simulink library "jud"  (Simulink 8.2)
settings: Solver=ode45  StartTime=0.0  StopTime=10.0  RelTol=1e-3
undefined symbols (not defined in the file or in its folder): ENUM_EPSADASABREASON_GEAR_POSITION_ERROR, ENUM_EPSADASABREASON_THERMAL_ERROR, ENUM_EPSADASABREASON_VEHICLE_SPEED_ERROR, ENUM_EPSLFCSTATUS_NOTAVAIL_PERM, ENUM_EPSLFCSTATUS_NOTAVAIL_TEMP, ENUM_EPSLFCSTATUS_OFF, ENUM_EPSLFCSTATUS_READY, ENUM_EPSLFCSTATUS_TRANSITION, ENUM_EPSLKASTATUS_NOTAVAIL_PERM, ENUM_EPSLKASTATUS_NOTAVAIL_TEMP, ENUM_EPSLKASTATUS_OFF, ENUM_EPSLKASTATUS_READY, ENUM_HMISTATE_ACTIVE, ENUM_KEYSWITCH_ON, ENUM_LFCSTATE_AUTOSTEERING, ENUM_LFCSTATE_STANDBY, ENUM_SENSORSTATE_NORMAL, FALSE, KAPP_VehicleWidth_m, KJUD_EPSLimition_kph, KJUD_EPSLimitionHysis_kph, KJUD_LFC4StandbyDelay_s, KJUD_SoftenTimerThr_s, TRUE, VJUD_LFCOffCount4LKAStandby_s, VJUD_LKAReActingDelay_s, VJUD_TLCTriggerReActingDelay_s
libraries: hcu_lib x12, simulink x10, jcc x1, jcw x1, jeb x1
(part 1 of 3)
settings Model: Creator=xsellart  LastModifiedBy=13192

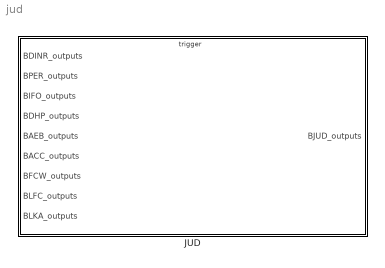
== system jud ==
  JUD : Subsystem

== system jud/JUD ==
  BDINR_outputs : Inport  OutDataTypeStr=Bus: BDINR_outputs
  BPER_outputs : Inport  Port=2  OutDataTypeStr=Bus: BPER_outputs
  BIFO_outputs : Inport  Port=3  OutDataTypeStr=Bus: BIFO_outputs
  BDHP_outputs : Inport  Port=4  OutDataTypeStr=Bus: BDHP_outputs
  BAEB_outputs : Inport  Port=5  OutDataTypeStr=Bus: BAEB_outputs
  BACC_outputs : Inport  Port=6  OutDataTypeStr=Bus: BACC_outputs
  BFCW_outputs : Inport  Port=7  OutDataTypeStr=Bus: BFCW_outputs
  BLFC_outputs : Inport  Port=8  OutDataTypeStr=Bus: BLFC_outputs
  BLKA_outputs : Inport  Port=9  OutDataTypeStr=Bus: BLKA_outputs
  trig_JUD : TriggerPort  TriggerType=function-call
      settings: AttributesFormatString=State = %<StatesWhenEnabling>
  Bus Creator : BusCreator  Inputs=61  OutDataTypeStr=Bus: BJUD_outputs
  jud : Subsystem
  BJUD_outputs : Outport  OutDataTypeStr=Bus: BJUD_outputs
  wires:
  Bus Creator/1 -> BJUD_outputs/1  "BJUD_outputs"
  BDINR_outputs/1 -> jud/1(BDINR_outputs)
  BPER_outputs/1 -> jud/2(BPER_outputs)
  BIFO_outputs/1 -> jud/3(BIFO_outputs)
  BDHP_outputs/1 -> jud/4(BDHP_outputs)
  BAEB_outputs/1 -> jud/5(BAEB_outputs)
  BACC_outputs/1 -> jud/6(BACC_outputs)
  BFCW_outputs/1 -> jud/7(BFCW_outputs)
  jud/1(VJUD_FCWEnableReq_flg) -> Bus Creator/1
  jud/2(VJUD_FCWOperational_flg) -> Bus Creator/2
  jud/8(VJUD_AEBEnableReq_flg) -> Bus Creator/8
  jud/41(VJUD_LKALeftActionReq_flg) -> Bus Creator/41
  jud/12(VJUD_AEBReturnOperational_flg) -> Bus Creator/12
  jud/31(VJUD_LFCTempFailureReq_flg) -> Bus Creator/31
  jud/10(VJUD_AEBSpeedInRange_flg) -> Bus Creator/10
  jud/20(VJUD_ACCOverrideReq_flg) -> Bus Creator/20
  jud/13(VJUD_AEBAutoBraking_flg) -> Bus Creator/13
  jud/11(VJUD_AEBActionReq_flg) -> Bus Creator/11
  jud/21(VJUD_ACCSetSpeed_kph) -> Bus Creator/21
  jud/34(VJUD_DegradedToAutoStr_flg) -> Bus Creator/34
  jud/44(VJUD_LKANoADASFailure_flg) -> Bus Creator/44
  jud/49(VJUD_LKATempFailureRecover_flg) -> Bus Creator/49
  jud/28(VJUD_LFCActionReq_flg) -> Bus Creator/28
  jud/33(VJUD_LFCOffRecover_flg) -> Bus Creator/33
  jud/42(VJUD_LKARightActionReq_flg) -> Bus Creator/42
  jud/29(VJUD_LFCDegradedReq_flg) -> Bus Creator/29
  jud/3(VJUD_FCWSpeedInRange_flg) -> Bus Creator/3
  jud/16(VJUD_ACCActiveReq_flg) -> Bus Creator/16
  jud/45(VJUD_LKAOffRecover_flg) -> Bus Creator/45
  jud/14(VJUD_AEBDeactivationReq_flg) -> Bus Creator/14
  jud/30(VJUD_LFCSoftenReq_flg) -> Bus Creator/30
  jud/26(VJUD_LFCCheckNormalFailure_flg) -> Bus Creator/26
  jud/15(VJUD_ACCEnableReq_flg) -> Bus Creator/15
  jud/7(VJUD_FCWDBSAllowed_flg) -> Bus Creator/7
  jud/47(VJUD_LKALeftOperationalRecover_flg) -> Bus Creator/47
  jud/24(VJUD_ACCSetSpeedSel_flg) -> Bus Creator/24
  jud/40(VJUD_LKAOperationalReq_flg) -> Bus Creator/40
  jud/5(VJUD_FCWReturnOperational_flg) -> Bus Creator/5
  jud/27(VJUD_LFCEnabledReq_flg) -> Bus Creator/27
  jud/43(VJUD_LKATempFailureReq_flg) -> Bus Creator/43
  jud/37(VJUD_LKACheckNormal_flg) -> Bus Creator/37
  jud/9(VJUD_AEBOperational_flg) -> Bus Creator/9
  jud/25(VJUD_LFCCheckNormal_flg) -> Bus Creator/25
  jud/39(VJUD_LKAEnabledReq_flg) -> Bus Creator/39
  jud/23(VJUD_ACCHMISelTimeGap_s) -> Bus Creator/23
  jud/17(VJUD_ACCDeactivationReq_flg) -> Bus Creator/17
  jud/36(VJUD_SoftenTimeThr_s) -> Bus Creator/36
  jud/46(VJUD_LKAStandbyRecover_flg) -> Bus Creator/46
  jud/4(VJUD_FCWActionReq_flg) -> Bus Creator/4
  jud/48(VJUD_LKARightOperationalRecover_flg) -> Bus Creator/48
  jud/22(VJUD_ACCSetTimeGap_s) -> Bus Creator/22
  jud/32(VJUD_LFCNoADASFailure_flg) -> Bus Creator/32
  jud/35(VJUD_LFCTempFailureRecover_flg) -> Bus Creator/35
  jud/18(VJUD_ACCStandstillReq_flg) -> Bus Creator/18
  jud/19(VJUD_ACCRefollowReq_flg) -> Bus Creator/19
  jud/38(VJUD_LKACheckNormalFailure_flg) -> Bus Creator/38
  BLFC_outputs/1 -> jud/8(BLFC_outputs)
  BLKA_outputs/1 -> jud/9(BLKA_outputs)
  jud/50(VJUD_LCACheckNormal_flg) -> Bus Creator/50
  jud/57(VJUD_LCAOffRecover_flg) -> Bus Creator/57
  jud/51(VJUD_LCAEnabledReq_flg) -> Bus Creator/51
  jud/56(VJUD_LCANoADASFailure_flg) -> Bus Creator/56
  jud/55(VJUD_LCATempFailureReq_flg) -> Bus Creator/55
  jud/58(VJUD_LCAStandbyRecover_flg) -> Bus Creator/58
  jud/59(VJUD_LCALeftOperationalRecover_flg) -> Bus Creator/59
  jud/52(VJUD_LCAOperationalReq_flg) -> Bus Creator/52
  jud/61(VJUD_LCATempFailureRecover_flg) -> Bus Creator/61
  jud/60(VJUD_LCARightOperationalRecover_flg) -> Bus Creator/60
  jud/53(VJUD_LCALeftActionReq_flg) -> Bus Creator/53
  jud/54(VJUD_LCARightActionReq_flg) -> Bus Creator/54
  jud/6(VJUD_FCWDeactivationReq_flg) -> Bus Creator/6

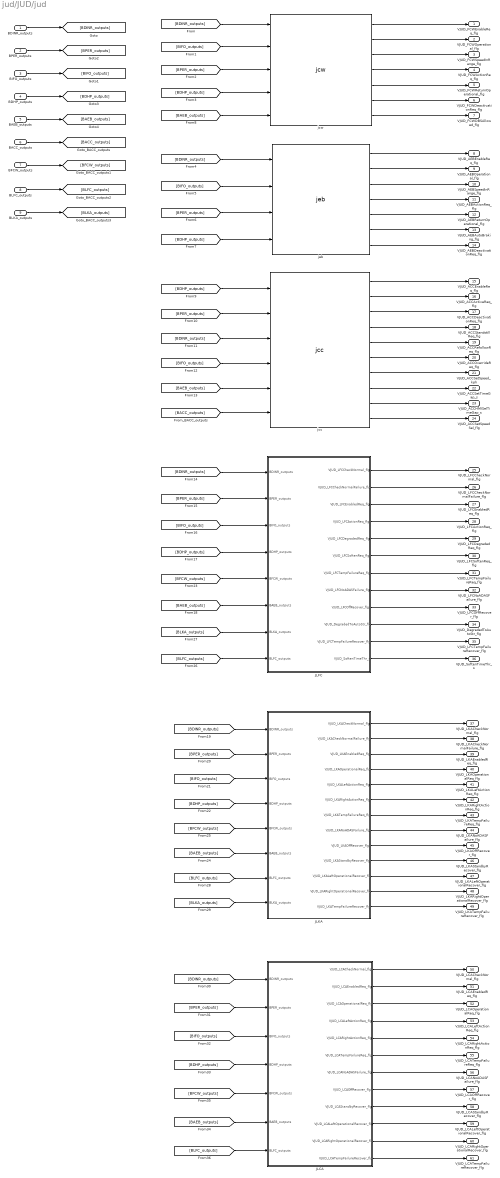
== system jud/JUD/jud ==
  BDINR_outputs : Inport  OutDataTypeStr=Bus: BDINR_outputs
  BPER_outputs : Inport  Port=2  OutDataTypeStr=Bus: BPER_outputs
  BIFO_outputs : Inport  Port=3  OutDataTypeStr=Bus: BIFO_outputs
  BDHP_outputs : Inport  Port=4  OutDataTypeStr=Bus: BDHP_outputs
  BAEB_outputs : Inport  Port=5  OutDataTypeStr=Bus: BAEB_outputs
  BACC_outputs : Inport  Port=6  OutDataTypeStr=Bus: BACC_outputs
  BFCW_outputs : Inport  Port=7  OutDataTypeStr=Bus: BFCW_outputs
  BLFC_outputs : Inport  Port=8  OutDataTypeStr=Bus: BLFC_outputs
  BLKA_outputs : Inport  Port=9  OutDataTypeStr=Bus: BLKA_outputs
  JLCA : Subsystem
  JLFC : Subsystem
  JLKA : Subsystem
  jcc : jcc/jcc
  jcw : jcw/jcw
  jeb : jeb/jeb
  VJUD_FCWEnableReq_flg : Outport
  VJUD_FCWOperational_flg : Outport  Port=2
  VJUD_FCWSpeedInRange_flg : Outport  Port=3
  VJUD_FCWActionReq_flg : Outport  Port=4
  VJUD_FCWReturnOperational_flg : Outport  Port=5
  VJUD_FCWDeactivationReq_flg : Outport  Port=6
  VJUD_FCWDBSAllowed_flg : Outport  Port=7
  VJUD_AEBEnableReq_flg : Outport  Port=8
  VJUD_AEBOperational_flg : Outport  Port=9
  VJUD_AEBSpeedInRange_flg : Outport  Port=10
  VJUD_AEBActionReq_flg : Outport  Port=11
  VJUD_AEBReturnOperational_flg : Outport  Port=12
  VJUD_AEBAutoBraking_flg : Outport  Port=13
  VJUD_AEBDeactivationReq_flg : Outport  Port=14
  VJUD_ACCEnableReq_flg : Outport  Port=15
  VJUD_ACCActiveReq_flg : Outport  Port=16
  VJUD_ACCDeactivationReq_flg : Outport  Port=17
  VJUD_ACCStandstillReq_flg : Outport  Port=18
  VJUD_ACCRefollowReq_flg : Outport  Port=19
  VJUD_ACCOverrideReq_flg : Outport  Port=20
  VJUD_ACCSetSpeed_kph : Outport  Port=21
  VJUD_ACCSetTimeGap_s : Outport  Port=22
  VJUD_ACCHMISelTimeGap_s : Outport  Port=23
  VJUD_ACCSetSpeedSel_flg : Outport  Port=24
  VJUD_LFCCheckNormal_flg : Outport  Port=25
  VJUD_LFCCheckNormalFailure_flg : Outport  Port=26
  VJUD_LFCEnabledReq_flg : Outport  Port=27
  VJUD_LFCActionReq_flg : Outport  Port=28
  VJUD_LFCDegradedReq_flg : Outport  Port=29
  VJUD_LFCSoftenReq_flg : Outport  Port=30
  VJUD_LFCTempFailureReq_flg : Outport  Port=31
  VJUD_LFCNoADASFailure_flg : Outport  Port=32
  VJUD_LFCOffRecover_flg : Outport  Port=33
  VJUD_DegradedToAutoStr_flg : Outport  Port=34
  VJUD_LFCTempFailureRecover_flg : Outport  Port=35
  VJUD_SoftenTimeThr_s : Outport  Port=36
  VJUD_LKACheckNormal_flg : Outport  Port=37
  VJUD_LKACheckNormalFailure_flg : Outport  Port=38
  VJUD_LKAEnabledReq_flg : Outport  Port=39
  VJUD_LKAOperationalReq_flg : Outport  Port=40
  VJUD_LKALeftActionReq_flg : Outport  Port=41
  VJUD_LKARightActionReq_flg : Outport  Port=42
  VJUD_LKATempFailureReq_flg : Outport  Port=43
  VJUD_LKANoADASFailure_flg : Outport  Port=44
  VJUD_LKAOffRecover_flg : Outport  Port=45
  VJUD_LKAStandbyRecover_flg : Outport  Port=46
  VJUD_LKALeftOperationalRecover_flg : Outport  Port=47
  VJUD_LKARightOperationalRecover_flg : Outport  Port=48
  VJUD_LKATempFailureRecover_flg : Outport  Port=49
  VJUD_LCACheckNormal_flg : Outport  Port=50
  VJUD_LCAEnabledReq_flg : Outport  Port=51
  VJUD_LCAOperationalReq_flg : Outport  Port=52
  VJUD_LCALeftActionReq_flg : Outport  Port=53
  VJUD_LCARightActionReq_flg : Outport  Port=54
  VJUD_LCATempFailureReq_flg : Outport  Port=55
  VJUD_LCANoADASFailure_flg : Outport  Port=56
  VJUD_LCAOffRecover_flg : Outport  Port=57
  VJUD_LCAStandbyRecover_flg : Outport  Port=58
  VJUD_LCALeftOperationalRecover_flg : Outport  Port=59
  VJUD_LCARightOperationalRecover_flg : Outport  Port=60
  VJUD_LCATempFailureRecover_flg : Outport  Port=61
  wires:
  [BIFO_outputs] -> jcw/2
  jeb/1 -> VJUD_AEBEnableReq_flg/1
  [BPER_outputs] -> jcw/3
  jcw/1 -> VJUD_FCWEnableReq_flg/1
  jcw/7 -> VJUD_FCWDBSAllowed_flg/1
  [BIFO_outputs] -> jeb/2
  [BDINR_outputs] -> jeb/1
  BPER_outputs/1 -> [BPER_outputs]
  jcw/6 -> VJUD_FCWDeactivationReq_flg/1
  jeb/6 -> VJUD_AEBAutoBraking_flg/1
  BIFO_outputs/1 -> [BIFO_outputs]
  BDHP_outputs/1 -> [BDHP_outputs]
  jcw/4 -> VJUD_FCWActionReq_flg/1
  [BDHP_outputs] -> jcw/4
  jcw/2 -> VJUD_FCWOperational_flg/1
  [BDHP_outputs] -> jeb/4
  jcw/3 -> VJUD_FCWSpeedInRange_flg/1
  jeb/4 -> VJUD_AEBActionReq_flg/1
  [BDINR_outputs] -> jcw/1
  [BPER_outputs] -> jeb/3
  BDINR_outputs/1 -> [BDINR_outputs]
  jeb/7 -> VJUD_AEBDeactivationReq_flg/1
  BAEB_outputs/1 -> [BAEB_outputs]
  [BAEB_outputs] -> jcw/5
  jeb/2 -> VJUD_AEBOperational_flg/1
  jeb/3 -> VJUD_AEBSpeedInRange_flg/1
  jcw/5 -> VJUD_FCWReturnOperational_flg/1
  jeb/5 -> VJUD_AEBReturnOperational_flg/1
  jcc/2 -> VJUD_ACCActiveReq_flg/1
  jcc/3 -> VJUD_ACCDeactivationReq_flg/1
  jcc/1 -> VJUD_ACCEnableReq_flg/1
  jcc/4 -> VJUD_ACCStandstillReq_flg/1
  jcc/5 -> VJUD_ACCRefollowReq_flg/1
  jcc/6 -> VJUD_ACCOverrideReq_flg/1
  jcc/7 -> VJUD_ACCSetSpeed_kph/1
  jcc/8 -> VJUD_ACCSetTimeGap_s/1
  jcc/10 -> VJUD_ACCSetSpeedSel_flg/1
  [BDHP_outputs] -> jcc/1
  [BPER_outputs] -> jcc/2
  [BDINR_outputs] -> jcc/3
  [BIFO_outputs] -> jcc/4
  [BAEB_outputs] -> jcc/5
  BACC_outputs/1 -> [BACC_outputs]
  [BACC_outputs] -> jcc/6
  jcc/9 -> VJUD_ACCHMISelTimeGap_s/1
  JLFC/1(VJUD_LFCCheckNormal_flg) -> VJUD_LFCCheckNormal_flg/1
  JLFC/2(VJUD_LFCCheckNormalFailure_flg) -> VJUD_LFCCheckNormalFailure_flg/1
  JLFC/3(VJUD_LFCEnabledReq_flg) -> VJUD_LFCEnabledReq_flg/1
  JLFC/4(VJUD_LFCActionReq_flg) -> VJUD_LFCActionReq_flg/1
  JLFC/5(VJUD_LFCDegradedReq_flg) -> VJUD_LFCDegradedReq_flg/1
  JLFC/6(VJUD_LFCSoftenReq_flg) -> VJUD_LFCSoftenReq_flg/1
  JLFC/7(VJUD_LFCTempFailureReq_flg) -> VJUD_LFCTempFailureReq_flg/1
  JLFC/8(VJUD_LFCNoADASFailure_flg) -> VJUD_LFCNoADASFailure_flg/1
  JLFC/9(VJUD_LFCOffRecover_flg) -> VJUD_LFCOffRecover_flg/1
  JLFC/10(VJUD_DegradedToAutoStr_flg) -> VJUD_DegradedToAutoStr_flg/1
  JLFC/11(VJUD_LFCTempFailureRecover_flg) -> VJUD_LFCTempFailureRecover_flg/1
  JLFC/12(VJUD_SoftenTimeThr_s) -> VJUD_SoftenTimeThr_s/1
  [BDINR_outputs] -> JLFC/1(BDINR_outputs)
  [BPER_outputs] -> JLFC/2(BPER_outputs)
  [BIFO_outputs] -> JLFC/3(BIFO_outputs)
  [BDHP_outputs] -> JLFC/4(BDHP_outputs)
  [BAEB_outputs] -> JLFC/6(BAEB_outputs)
  BFCW_outputs/1 -> [BFCW_outputs]
  [BPER_outputs] -> JLKA/2(BPER_outputs)
  [BDINR_outputs] -> JLKA/1(BDINR_outputs)
  [BIFO_outputs] -> JLKA/3(BIFO_outputs)
  [BDHP_outputs] -> JLKA/4(BDHP_outputs)
  [BFCW_outputs] -> JLFC/5(BFCW_outputs)
  [BAEB_outputs] -> JLKA/6(BAEB_outputs)
  [BFCW_outputs] -> JLKA/5(BFCW_outputs)
  JLKA/1(VJUD_LKACheckNormal_flg) -> VJUD_LKACheckNormal_flg/1
  JLKA/2(VJUD_LKACheckNormalFailure_flg) -> VJUD_LKACheckNormalFailure_flg/1
  JLKA/3(VJUD_LKAEnabledReq_flg) -> VJUD_LKAEnabledReq_flg/1
  JLKA/4(VJUD_LKAOperationalReq_flg) -> VJUD_LKAOperationalReq_flg/1
  JLKA/5(VJUD_LKALeftActionReq_flg) -> VJUD_LKALeftActionReq_flg/1
  JLKA/6(VJUD_LKARightActionReq_flg) -> VJUD_LKARightActionReq_flg/1
  JLKA/7(VJUD_LKATempFailureReq_flg) -> VJUD_LKATempFailureReq_flg/1
  JLKA/8(VJUD_LKANoADASFailure_flg) -> VJUD_LKANoADASFailure_flg/1
  JLKA/9(VJUD_LKAOffRecover_flg) -> VJUD_LKAOffRecover_flg/1
  JLKA/10(VJUD_LKAStandbyRecover_flg) -> VJUD_LKAStandbyRecover_flg/1
  JLKA/11(VJUD_LKALeftOperationalRecover_flg) -> VJUD_LKALeftOperationalRecover_flg/1
  JLKA/12(VJUD_LKARightOperationalRecover_flg) -> VJUD_LKARightOperationalRecover_flg/1
  JLKA/13(VJUD_LKATempFailureRecover_flg) -> VJUD_LKATempFailureRecover_flg/1
  BLFC_outputs/1 -> [BLFC_outputs]
  BLKA_outputs/1 -> [BLKA_outputs]
  [BLKA_outputs] -> JLKA/8(BLKA_outputs)
  [BLFC_outputs] -> JLKA/7(BLFC_outputs)
  [BLKA_outputs] -> JLFC/7(BLKA_outputs)
  [BLFC_outputs] -> JLFC/8(BLFC_outputs)
  [BDINR_outputs] -> JLCA/1(BDINR_outputs)
  [BPER_outputs] -> JLCA/2(BPER_outputs)
  [BIFO_outputs] -> JLCA/3(BIFO_outputs)
  [BDHP_outputs] -> JLCA/4(BDHP_outputs)
  [BFCW_outputs] -> JLCA/5(BFCW_outputs)
  [BAEB_outputs] -> JLCA/6(BAEB_outputs)
  [BLFC_outputs] -> JLCA/7(BLFC_outputs)
  JLCA/1(VJUD_LCACheckNormal_flg) -> VJUD_LCACheckNormal_flg/1
  JLCA/2(VJUD_LCAEnabledReq_flg) -> VJUD_LCAEnabledReq_flg/1
  JLCA/3(VJUD_LCAOperationalReq_flg) -> VJUD_LCAOperationalReq_flg/1
  JLCA/4(VJUD_LCALeftActionReq_flg) -> VJUD_LCALeftActionReq_flg/1
  JLCA/5(VJUD_LCARightActionReq_flg) -> VJUD_LCARightActionReq_flg/1
  JLCA/6(VJUD_LCATempFailureReq_flg) -> VJUD_LCATempFailureReq_flg/1
  JLCA/7(VJUD_LCANoADASFailure_flg) -> VJUD_LCANoADASFailure_flg/1
  JLCA/8(VJUD_LCAOffRecover_flg) -> VJUD_LCAOffRecover_flg/1
  JLCA/9(VJUD_LCAStandbyRecover_flg) -> VJUD_LCAStandbyRecover_flg/1
  JLCA/10(VJUD_LCALeftOperationalRecover_flg) -> VJUD_LCALeftOperationalRecover_flg/1
  JLCA/11(VJUD_LCARightOperationalRecover_flg) -> VJUD_LCARightOperationalRecover_flg/1
  JLCA/12(VJUD_LCATempFailureRecover_flg) -> VJUD_LCATempFailureRecover_flg/1

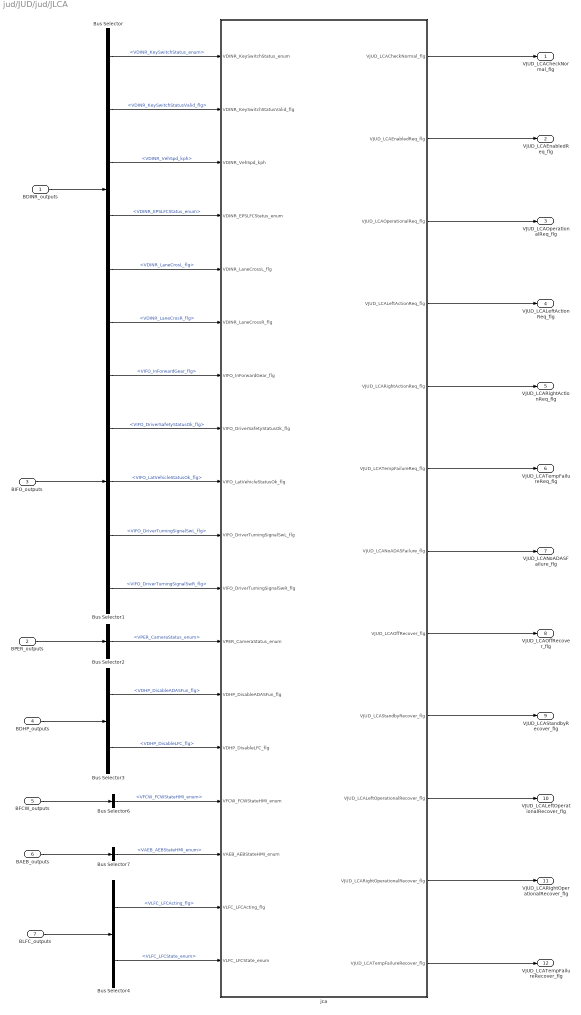
== system jud/JUD/jud/JLCA ==
  BDINR_outputs : Inport  OutDataTypeStr=Bus: BDINR_outputs
  BPER_outputs : Inport  Port=2  OutDataTypeStr=Bus: BPER_outputs
  BIFO_outputs : Inport  Port=3  OutDataTypeStr=Bus: BIFO_outputs
  BDHP_outputs : Inport  Port=4  OutDataTypeStr=Bus: BDHP_outputs
  BFCW_outputs : Inport  Port=5  OutDataTypeStr=Bus: BFCW_outputs
  BAEB_outputs : Inport  Port=6  OutDataTypeStr=Bus: BAEB_outputs
  BLFC_outputs : Inport  Port=7  OutDataTypeStr=Bus: BLFC_outputs
  Bus Selector : BusSelector  OutputSignals=VDINR_KeySwitchStatus_enum,VDINR_KeySwitchStatusValid_flg,VDINR_VehSpd_kph,VDINR_EPSLFCStatus_enum,VDINR_LaneCrosL_flg,VDINR_LaneCrosR_flg
  Bus Selector1 : BusSelector  OutputSignals=VIFO_InForwardGear_flg,VIFO_DriverSafetyStatusOk_flg,VIFO_LatVehicleStatusOk_flg,VIFO_DriverTurningSignalSwL_flg,VIFO_DriverTurningSignalSwR_flg
  Bus Selector2 : BusSelector  OutputSignals=VPER_CameraStatus_enum
  Bus Selector3 : BusSelector  OutputSignals=VDHP_DisableADASFun_flg,VDHP_DisableLFC_flg
  Bus Selector4 : BusSelector  OutputSignals=VLFC_LFCActing_flg,VLFC_LFCState_enum
  Bus Selector6 : BusSelector  OutputSignals=VFCW_FCWStateHMI_enum
  Bus Selector7 : BusSelector  OutputSignals=VAEB_AEBStateHMI_enum
  jca : Subsystem
  VJUD_LCACheckNormal_flg : Outport
  VJUD_LCAEnabledReq_flg : Outport  Port=2
  VJUD_LCAOperationalReq_flg : Outport  Port=3
  VJUD_LCALeftActionReq_flg : Outport  Port=4
  VJUD_LCARightActionReq_flg : Outport  Port=5
  VJUD_LCATempFailureReq_flg : Outport  Port=6
  VJUD_LCANoADASFailure_flg : Outport  Port=7
  VJUD_LCAOffRecover_flg : Outport  Port=8
  VJUD_LCAStandbyRecover_flg : Outport  Port=9
  VJUD_LCALeftOperationalRecover_flg : Outport  Port=10
  VJUD_LCARightOperationalRecover_flg : Outport  Port=11
  VJUD_LCATempFailureRecover_flg : Outport  Port=12
  wires:
  jca/1(VJUD_LCACheckNormal_flg) -> VJUD_LCACheckNormal_flg/1
  jca/2(VJUD_LCAEnabledReq_flg) -> VJUD_LCAEnabledReq_flg/1
  jca/3(VJUD_LCAOperationalReq_flg) -> VJUD_LCAOperationalReq_flg/1
  jca/4(VJUD_LCALeftActionReq_flg) -> VJUD_LCALeftActionReq_flg/1
  jca/6(VJUD_LCATempFailureReq_flg) -> VJUD_LCATempFailureReq_flg/1
  jca/7(VJUD_LCANoADASFailure_flg) -> VJUD_LCANoADASFailure_flg/1
  jca/8(VJUD_LCAOffRecover_flg) -> VJUD_LCAOffRecover_flg/1
  jca/9(VJUD_LCAStandbyRecover_flg) -> VJUD_LCAStandbyRecover_flg/1
  jca/10(VJUD_LCALeftOperationalRecover_flg) -> VJUD_LCALeftOperationalRecover_flg/1
  jca/12(VJUD_LCATempFailureRecover_flg) -> VJUD_LCATempFailureRecover_flg/1
  jca/5(VJUD_LCARightActionReq_flg) -> VJUD_LCARightActionReq_flg/1
  BPER_outputs/1 -> Bus Selector2/1
  BIFO_outputs/1 -> Bus Selector1/1
  BDHP_outputs/1 -> Bus Selector3/1
  BDINR_outputs/1 -> Bus Selector/1
  BLFC_outputs/1 -> Bus Selector4/1
  jca/11(VJUD_LCARightOperationalRecover_flg) -> VJUD_LCARightOperationalRecover_flg/1
  BFCW_outputs/1 -> Bus Selector6/1
  BAEB_outputs/1 -> Bus Selector7/1
  Bus Selector3/2 -> jca/14(VDHP_DisableLFC_flg)  "<VDHP_DisableLFC_flg>"
  Bus Selector6/1 -> jca/15(VFCW_FCWStateHMI_enum)  "<VFCW_FCWStateHMI_enum>"
  Bus Selector7/1 -> jca/16(VAEB_AEBStateHMI_enum)  "<VAEB_AEBStateHMI_enum>"
  Bus Selector4/1 -> jca/17(VLFC_LFCActing_flg)  "<VLFC_LFCActing_flg>"
  Bus Selector4/2 -> jca/18(VLFC_LFCState_enum)  "<VLFC_LFCState_enum>"
  Bus Selector/1 -> jca/1(VDINR_KeySwitchStatus_enum)  "<VDINR_KeySwitchStatus_enum>"
  Bus Selector/2 -> jca/2(VDINR_KeySwitchStatusValid_flg)  "<VDINR_KeySwitchStatusValid_flg>"
  Bus Selector/3 -> jca/3(VDINR_VehSpd_kph)  "<VDINR_VehSpd_kph>"
  Bus Selector/4 -> jca/4(VDINR_EPSLFCStatus_enum)  "<VDINR_EPSLFCStatus_enum>"
  Bus Selector/5 -> jca/5(VDINR_LaneCrossL_flg)  "<VDINR_LaneCrosL_flg>"
  Bus Selector/6 -> jca/6(VDINR_LaneCrossR_flg)  "<VDINR_LaneCrosR_flg>"
  Bus Selector1/1 -> jca/7(VIFO_InForwardGear_flg)  "<VIFO_InForwardGear_flg>"
  Bus Selector1/2 -> jca/8(VIFO_DriverSafetyStatusOk_flg)  "<VIFO_DriverSafetyStatusOk_flg>"
  Bus Selector1/3 -> jca/9(VIFO_LatVehicleStatusOk_flg)  "<VIFO_LatVehicleStatusOk_flg>"
  Bus Selector2/1 -> jca/12(VPER_CameraStatus_enum)  "<VPER_CameraStatus_enum>"
  Bus Selector3/1 -> jca/13(VDHP_DisableADASFun_flg)  "<VDHP_DisableADASFun_flg>"
  Bus Selector1/4 -> jca/10(VIFO_DriverTurningSignalSwL_flg)  "<VIFO_DriverTurningSignalSwL_flg>"
  Bus Selector1/5 -> jca/11(VIFO_DriverTurningSignalSwR_flg)  "<VIFO_DriverTurningSignalSwR_flg>"

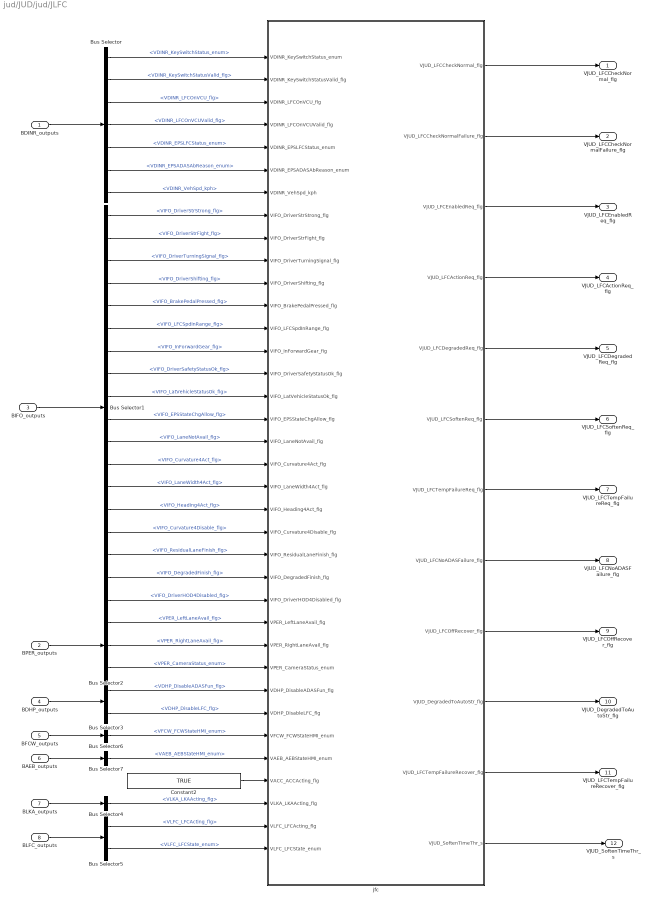
== system jud/JUD/jud/JLFC ==
  BDINR_outputs : Inport  OutDataTypeStr=Bus: BDINR_outputs
  BPER_outputs : Inport  Port=2  OutDataTypeStr=Bus: BPER_outputs
  BIFO_outputs : Inport  Port=3  OutDataTypeStr=Bus: BIFO_outputs
  BDHP_outputs : Inport  Port=4  OutDataTypeStr=Bus: BDHP_outputs
  BFCW_outputs : Inport  Port=5  OutDataTypeStr=Bus: BFCW_outputs
  BAEB_outputs : Inport  Port=6  OutDataTypeStr=Bus: BAEB_outputs
  BLKA_outputs : Inport  Port=7  OutDataTypeStr=Bus: BLKA_outputs
  BLFC_outputs : Inport  Port=8  OutDataTypeStr=Bus: BLFC_outputs
  Bus Selector : BusSelector  OutputSignals=VDINR_KeySwitchStatus_enum,VDINR_KeySwitchStatusValid_flg,VDINR_LFCOnVCU_flg,VDINR_LFCOnVCUValid_flg,VDINR_EPSLFCStatus_enum,VDINR_EPSADASAbReason_enum,VDINR_VehSpd_kph
  Bus Selector1 : BusSelector  OutputSignals=VIFO_DriverStrStrong_flg,VIFO_DriverStrFight_flg,VIFO_DriverTurningSignal_flg,VIFO_DriverShifting_flg,VIFO_BrakePedalPressed_flg,VIFO_LFCSpdInRange_flg,VIFO_InForwardGear_flg,VIFO_DriverSafetyStatusOk_flg,VIFO_LatVehicleStatusOk_flg,VIFO_EPSStateChgAllow_flg,VIFO_LaneNotAvail_flg,VIFO_Curvature4Act_flg,VIFO_LaneWidth4Act_flg,VIFO_Heading4Act_flg,VIFO_Curvature4Disable_flg,VIFO_ResidualLaneFinish_flg,VIFO_DegradedFinish_flg,VIFO_DriverHOD4Disabled_flg
  Bus Selector2 : BusSelector  OutputSignals=VPER_LeftLaneAvail_flg,VPER_RightLaneAvail_flg,VPER_CameraStatus_enum
  Bus Selector3 : BusSelector  OutputSignals=VDHP_DisableADASFun_flg,VDHP_DisableLFC_flg
  Bus Selector4 : BusSelector  OutputSignals=VLKA_LKAActing_flg
  Bus Selector5 : BusSelector  OutputSignals=VLFC_LFCActing_flg,VLFC_LFCState_enum
  Bus Selector6 : BusSelector  OutputSignals=VFCW_FCWStateHMI_enum
  Bus Selector7 : BusSelector  OutputSignals=VAEB_AEBStateHMI_enum
  Constant2 : Constant  Value=TRUE
  jfc : Subsystem
  VJUD_LFCCheckNormal_flg : Outport
  VJUD_LFCCheckNormalFailure_flg : Outport  Port=2
  VJUD_LFCEnabledReq_flg : Outport  Port=3
  VJUD_LFCActionReq_flg : Outport  Port=4
  VJUD_LFCDegradedReq_flg : Outport  Port=5
  VJUD_LFCSoftenReq_flg : Outport  Port=6
  VJUD_LFCTempFailureReq_flg : Outport  Port=7
  VJUD_LFCNoADASFailure_flg : Outport  Port=8
  VJUD_LFCOffRecover_flg : Outport  Port=9
  VJUD_DegradedToAutoStr_flg : Outport  Port=10
  VJUD_LFCTempFailureRecover_flg : Outport  Port=11
  VJUD_SoftenTimeThr_s : Outport  Port=12
  wires:
  BPER_outputs/1 -> Bus Selector2/1
  BIFO_outputs/1 -> Bus Selector1/1
  BDHP_outputs/1 -> Bus Selector3/1
  BDINR_outputs/1 -> Bus Selector/1
  BLKA_outputs/1 -> Bus Selector4/1
  BLFC_outputs/1 -> Bus Selector5/1
  jfc/1(VJUD_LFCCheckNormal_flg) -> VJUD_LFCCheckNormal_flg/1
  jfc/11(VJUD_LFCTempFailureRecover_flg) -> VJUD_LFCTempFailureRecover_flg/1
  jfc/12(VJUD_SoftenTimeThr_s) -> VJUD_SoftenTimeThr_s/1
  Bus Selector6/1 -> jfc/31(VFCW_FCWStateHMI_enum)  "<VFCW_FCWStateHMI_enum>"
  Constant2/1 -> jfc/33(VACC_ACCActing_flg)
  Bus Selector4/1 -> jfc/34(VLKA_LKAActing_flg)  "<VLKA_LKAActing_flg>"
  Bus Selector5/1 -> jfc/35(VLFC_LFCActing_flg)  "<VLFC_LFCActing_flg>"
  Bus Selector/2 -> jfc/2(VDINR_KeySwitchStatusValid_flg)  "<VDINR_KeySwitchStatusValid_flg>"
  Bus Selector/1 -> jfc/1(VDINR_KeySwitchStatus_enum)  "<VDINR_KeySwitchStatus_enum>"
  Bus Selector/3 -> jfc/3(VDINR_LFCOnVCU_flg)  "<VDINR_LFCOnVCU_flg>"
  Bus Selector/4 -> jfc/4(VDINR_LFCOnVCUValid_flg)  "<VDINR_LFCOnVCUValid_flg>"
  Bus Selector/5 -> jfc/5(VDINR_EPSLFCStatus_enum)  "<VDINR_EPSLFCStatus_enum>"
  Bus Selector/6 -> jfc/6(VDINR_EPSADASAbReason_enum)  "<VDINR_EPSADASAbReason_enum>"
  Bus Selector/7 -> jfc/7(VDINR_VehSpd_kph)  "<VDINR_VehSpd_kph>"
  Bus Selector1/1 -> jfc/8(VIFO_DriverStrStrong_flg)  "<VIFO_DriverStrStrong_flg>"
  Bus Selector1/2 -> jfc/9(VIFO_DriverStrFight_flg)  "<VIFO_DriverStrFight_flg>"
  Bus Selector1/3 -> jfc/10(VIFO_DriverTurningSignal_flg)  "<VIFO_DriverTurningSignal_flg>"
  Bus Selector2/3 -> jfc/28(VPER_CameraStatus_enum)  "<VPER_CameraStatus_enum>"
  Bus Selector3/1 -> jfc/29(VDHP_DisableADASFun_flg)  "<VDHP_DisableADASFun_flg>"
  Bus Selector3/2 -> jfc/30(VDHP_DisableLFC_flg)  "<VDHP_DisableLFC_flg>"
  Bus Selector2/2 -> jfc/27(VPER_RightLaneAvail_flg)  "<VPER_RightLaneAvail_flg>"
  BFCW_outputs/1 -> Bus Selector6/1
  Bus Selector7/1 -> jfc/32(VAEB_AEBStateHMI_enum)  "<VAEB_AEBStateHMI_enum>"
  BAEB_outputs/1 -> Bus Selector7/1
  Bus Selector5/2 -> jfc/36(VLFC_LFCState_enum)  "<VLFC_LFCState_enum>"
  Bus Selector1/4 -> jfc/11(VIFO_DriverShifting_flg)  "<VIFO_DriverShifting_flg>"
  Bus Selector1/5 -> jfc/12(VIFO_BrakePedalPressed_flg)  "<VIFO_BrakePedalPressed_flg>"
  Bus Selector1/6 -> jfc/13("VIFO_LFCSpdInRange_flg ")  "<VIFO_LFCSpdInRange_flg>"
  Bus Selector1/7 -> jfc/14(VIFO_InForwardGear_fig)  "<VIFO_InForwardGear_flg>"
  Bus Selector1/8 -> jfc/15(VIFO_DriverSafetyStatusOk_flg)  "<VIFO_DriverSafetyStatusOk_flg>"
  Bus Selector1/9 -> jfc/16(VIFO_LatVehicleStatusOk_flg)  "<VIFO_LatVehicleStatusOk_flg>"
  Bus Selector1/10 -> jfc/17(VIFO_EPSStateChgAllow_flg)  "<VIFO_EPSStateChgAllow_flg>"
  Bus Selector1/11 -> jfc/18(VIFO_LaneNotAvail_fig)  "<VIFO_LaneNotAvail_flg>"
  Bus Selector1/12 -> jfc/19(VIFO_Curvature4Act_flg)  "<VIFO_Curvature4Act_flg>"
  Bus Selector1/13 -> jfc/20(VIFO_LaneWidth4Act_flg)  "<VIFO_LaneWidth4Act_flg>"
  Bus Selector1/14 -> jfc/21(VIFO_Heading4Act_flg)  "<VIFO_Heading4Act_flg>"
  Bus Selector1/15 -> jfc/22(VIFO_Curvature4Disable_flg)  "<VIFO_Curvature4Disable_flg>"
  Bus Selector1/16 -> jfc/23(VIFO_ResidualLaneFinish_flg)  "<VIFO_ResidualLaneFinish_flg>"
  Bus Selector1/17 -> jfc/24(VIFO_DegradedFinish_flg)  "<VIFO_DegradedFinish_flg>"
  Bus Selector1/18 -> jfc/25(VIFO_DriverHOD4Disabled_flg)  "<VIFO_DriverHOD4Disabled_flg>"
  Bus Selector2/1 -> jfc/26(VPER_LeftLaneAvail_flg)  "<VPER_LeftLaneAvail_flg>"
  jfc/10(VJUD_DegradedToAutoStr_flg) -> VJUD_DegradedToAutoStr_flg/1
  jfc/9(VJUD_LFCOffRecover_flg) -> VJUD_LFCOffRecover_flg/1
  jfc/8(VJUD_LFCNoADASFailure_flg) -> VJUD_LFCNoADASFailure_flg/1
  jfc/7(VJUD_LFCTempFailureReq_flg) -> VJUD_LFCTempFailureReq_flg/1
  jfc/6(VJUD_LFCSoftenReq_flg) -> VJUD_LFCSoftenReq_flg/1
  jfc/5(VJUD_LFCDegradedReq_flg) -> VJUD_LFCDegradedReq_flg/1
  jfc/4(VJUD_LFCActionReq_flg) -> VJUD_LFCActionReq_flg/1
  jfc/3(VJUD_LFCEnabledReq_flg) -> VJUD_LFCEnabledReq_flg/1
  jfc/2(VJUD_LFCCheckNormalFailure_flg) -> VJUD_LFCCheckNormalFailure_flg/1

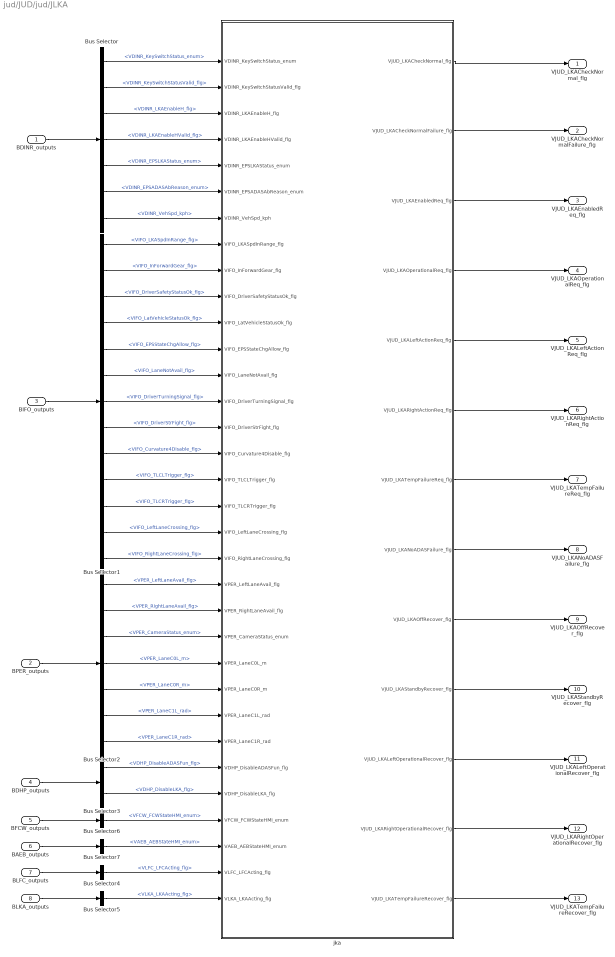
== system jud/JUD/jud/JLKA ==
  BDINR_outputs : Inport  OutDataTypeStr=Bus: BDINR_outputs
  BPER_outputs : Inport  Port=2  OutDataTypeStr=Bus: BPER_outputs
  BIFO_outputs : Inport  Port=3  OutDataTypeStr=Bus: BIFO_outputs
  BDHP_outputs : Inport  Port=4  OutDataTypeStr=Bus: BDHP_outputs
  BFCW_outputs : Inport  Port=5  OutDataTypeStr=Bus: BFCW_outputs
  BAEB_outputs : Inport  Port=6  OutDataTypeStr=Bus: BAEB_outputs
  BLFC_outputs : Inport  Port=7  OutDataTypeStr=Bus: BLFC_outputs
  BLKA_outputs : Inport  Port=8  OutDataTypeStr=Bus: BLKA_outputs
  Bus Selector : BusSelector  OutputSignals=VDINR_KeySwitchStatus_enum,VDINR_KeySwitchStatusValid_flg,VDINR_LKAEnableH_flg,VDINR_LKAEnableHValid_flg,VDINR_EPSLKAStatus_enum,VDINR_EPSADASAbReason_enum,VDINR_VehSpd_kph
  Bus Selector1 : BusSelector  OutputSignals=VIFO_LKASpdInRange_flg,VIFO_InForwardGear_flg,VIFO_DriverSafetyStatusOk_flg,VIFO_LatVehicleStatusOk_flg,VIFO_EPSStateChgAllow_flg,VIFO_LaneNotAvail_flg,VIFO_DriverTurningSignal_flg,VIFO_DriverStrFight_flg,VIFO_Curvature4Disable_flg,VIFO_TLCLTrigger_flg,VIFO_TLCRTrigger_flg,VIFO_LeftLaneCrossing_flg,VIFO_RightLaneCrossing_flg
  Bus Selector2 : BusSelector  OutputSignals=VPER_LeftLaneAvail_flg,VPER_RightLaneAvail_flg,VPER_CameraStatus_enum,VPER_LaneC0L_m,VPER_LaneC0R_m,VPER_LaneC1L_rad,VPER_LaneC1R_rad
  Bus Selector3 : BusSelector  OutputSignals=VDHP_DisableADASFun_flg,VDHP_DisableLKA_flg
  Bus Selector4 : BusSelector  OutputSignals=VLFC_LFCActing_flg
  Bus Selector5 : BusSelector  OutputSignals=VLKA_LKAActing_flg
  Bus Selector6 : BusSelector  OutputSignals=VFCW_FCWStateHMI_enum
  Bus Selector7 : BusSelector  OutputSignals=VAEB_AEBStateHMI_enum
  jka : Subsystem
  VJUD_LKACheckNormal_flg : Outport
  VJUD_LKACheckNormalFailure_flg : Outport  Port=2
  VJUD_LKAEnabledReq_flg : Outport  Port=3
  VJUD_LKAOperationalReq_flg : Outport  Port=4
  VJUD_LKALeftActionReq_flg : Outport  Port=5
  VJUD_LKARightActionReq_flg : Outport  Port=6
  VJUD_LKATempFailureReq_flg : Outport  Port=7
  VJUD_LKANoADASFailure_flg : Outport  Port=8
  VJUD_LKAOffRecover_flg : Outport  Port=9
  VJUD_LKAStandbyRecover_flg : Outport  Port=10
  VJUD_LKALeftOperationalRecover_flg : Outport  Port=11
  VJUD_LKARightOperationalRecover_flg : Outport  Port=12
  VJUD_LKATempFailureRecover_flg : Outport  Port=13
  wires:
  jka/1(VJUD_LKACheckNormal_flg) -> VJUD_LKACheckNormal_flg/1
  jka/3(VJUD_LKAEnabledReq_flg) -> VJUD_LKAEnabledReq_flg/1
  jka/4(VJUD_LKAOperationalReq_flg) -> VJUD_LKAOperationalReq_flg/1
  jka/5(VJUD_LKALeftActionReq_flg) -> VJUD_LKALeftActionReq_flg/1
  jka/7(VJUD_LKATempFailureReq_flg) -> VJUD_LKATempFailureReq_flg/1
  jka/8(VJUD_LKANoADASFailure_flg) -> VJUD_LKANoADASFailure_flg/1
  jka/9(VJUD_LKAOffRecover_flg) -> VJUD_LKAOffRecover_flg/1
  jka/10(VJUD_LKAStandbyRecover_flg) -> VJUD_LKAStandbyRecover_flg/1
  jka/11(VJUD_LKALeftOperationalRecover_flg) -> VJUD_LKALeftOperationalRecover_flg/1
  jka/13(VJUD_LKATempFailureRecover_flg) -> VJUD_LKATempFailureRecover_flg/1
  jka/6(VJUD_LKARightActionReq_flg) -> VJUD_LKARightActionReq_flg/1
  BPER_outputs/1 -> Bus Selector2/1
  BIFO_outputs/1 -> Bus Selector1/1
  BDHP_outputs/1 -> Bus Selector3/1
  BDINR_outputs/1 -> Bus Selector/1
  Bus Selector/6 -> jka/6(VDINR_EPSADASAbReason_enum)  "<VDINR_EPSADASAbReason_enum>"
  Bus Selector/2 -> jka/2(VDINR_KeySwitchStatusValid_flg)  "<VDINR_KeySwitchStatusValid_flg>"
  Bus Selector/7 -> jka/7(VDINR_VehSpd_kph)  "<VDINR_VehSpd_kph>"
  Bus Selector/5 -> jka/5(VDINR_EPSLKAStatus_enum)  "<VDINR_EPSLKAStatus_enum>"
  Bus Selector/1 -> jka/1(VDINR_KeySwitchStatus_enum)  "<VDINR_KeySwitchStatus_enum>"
  Bus Selector/4 -> jka/4(VDINR_LKAEnableHValid_flg)  "<VDINR_LKAEnableHValid_flg>"
  Bus Selector/3 -> jka/3(VDINR_LKAEnableH_flg)  "<VDINR_LKAEnableH_flg>"
  Bus Selector1/1 -> jka/8("VIFO_LKASpdInRange_flg ")  "<VIFO_LKASpdInRange_flg>"
  Bus Selector1/2 -> jka/9(VIFO_InForwardGear_flg)  "<VIFO_InForwardGear_flg>"
  Bus Selector1/3 -> jka/10(VIFO_DriverSafetyStatusOk_flg)  "<VIFO_DriverSafetyStatusOk_flg>"
  Bus Selector1/4 -> jka/11(VIFO_LatVehicleStatusOk_flg)  "<VIFO_LatVehicleStatusOk_flg>"
  Bus Selector1/5 -> jka/12(VIFO_EPSStateChgAllow_flg)  "<VIFO_EPSStateChgAllow_flg>"
  Bus Selector1/6 -> jka/13(VIFO_LaneNotAvail_flg)  "<VIFO_LaneNotAvail_flg>"
  Bus Selector1/7 -> jka/14(VIFO_DriverTurningSignal_flg)  "<VIFO_DriverTurningSignal_flg>"
  Bus Selector1/8 -> jka/15(VIFO_DriverStrFight_flg)  "<VIFO_DriverStrFight_flg>"
  Bus Selector1/9 -> jka/16(VIFO_Curvature4Disable_flg)  "<VIFO_Curvature4Disable_flg>"
  Bus Selector1/10 -> jka/17(VIFO_TLCLTrigger_flg)  "<VIFO_TLCLTrigger_flg>"
  Bus Selector1/11 -> jka/18(VIFO_TLCRTrigger_flg)  "<VIFO_TLCRTrigger_flg>"
  Bus Selector2/3 -> jka/23(VPER_CameraStatus_enum)  "<VPER_CameraStatus_enum>"
  Bus Selector2/1 -> jka/21(VPER_LeftLaneAvail_flg)  "<VPER_LeftLaneAvail_flg>"
  Bus Selector2/2 -> jka/22(VPER_RightLaneAvail_flg)  "<VPER_RightLaneAvail_flg>"
  Bus Selector3/1 -> jka/28(VDHP_DisableADASFun_flg)  "<VDHP_DisableADASFun_flg>"
  Bus Selector3/2 -> jka/29(VDHP_DisableLKA_flg)  "<VDHP_DisableLKA_flg>"
  BLFC_outputs/1 -> Bus Selector4/1
  Bus Selector4/1 -> jka/32(VLFC_LFCActing_flg)  "<VLFC_LFCActing_flg>"
  jka/12(VJUD_LKARightOperationalRecover_flg) -> VJUD_LKARightOperationalRecover_flg/1
  Bus Selector2/4 -> jka/24(VPER_LaneC0L_m)  "<VPER_LaneC0L_m>"
  Bus Selector2/5 -> jka/25(VPER_LaneC0R_m)  "<VPER_LaneC0R_m>"
  Bus Selector2/6 -> jka/26(VPER_LaneC1L_rad)  "<VPER_LaneC1L_rad>"
  Bus Selector2/7 -> jka/27(VPER_LaneC1R_rad)  "<VPER_LaneC1R_rad>"
  Bus Selector1/12 -> jka/19(VIFO_LeftLaneCrossing_flg)  "<VIFO_LeftLaneCrossing_flg>"
  Bus Selector1/13 -> jka/20(VIFO_RightLaneCrossing_flg)  "<VIFO_RightLaneCrossing_flg>"
  BFCW_outputs/1 -> Bus Selector6/1
  BAEB_outputs/1 -> Bus Selector7/1
  Bus Selector6/1 -> jka/30(VFCW_FCWStateHMI_enum)  "<VFCW_FCWStateHMI_enum>"
  Bus Selector7/1 -> jka/31(VAEB_AEBStateHMI_enum)  "<VAEB_AEBStateHMI_enum>"
  BLKA_outputs/1 -> Bus Selector5/1
  Bus Selector5/1 -> jka/33(VLKA_LKAActing_flg)  "<VLKA_LKAActing_flg>"
  jka/2(VJUD_LKACheckNormalFailure_flg) -> VJUD_LKACheckNormalFailure_flg/1

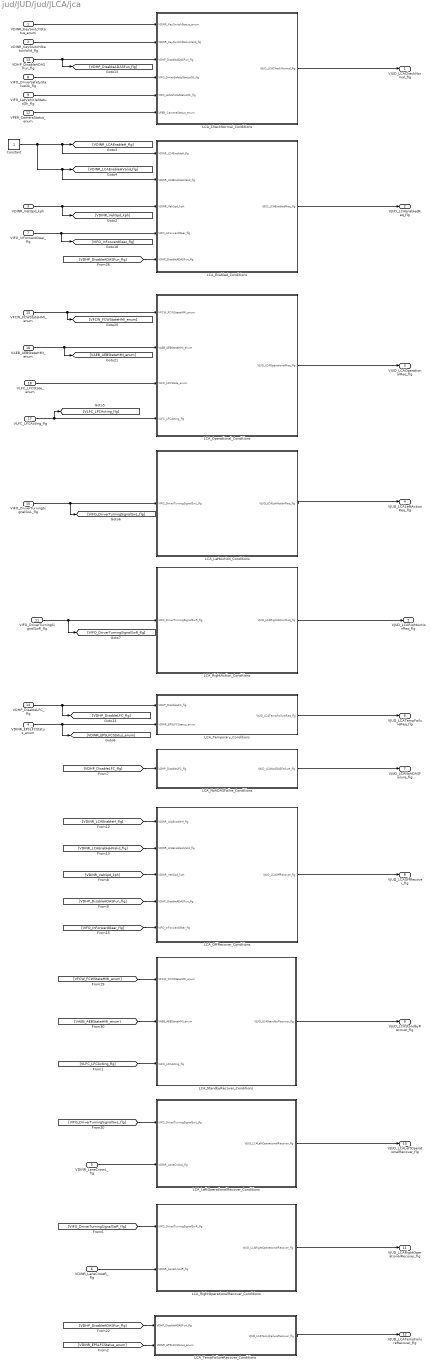
== system jud/JUD/jud/JLCA/jca ==
  VDINR_KeySwitchStatus_enum : Inport
  VDINR_KeySwitchStatusValid_flg : Inport  Port=2
  VDINR_VehSpd_kph : Inport  Port=3
  VDINR_EPSLFCStatus_enum : Inport  Port=4
  VDINR_LaneCrossL_flg : Inport  Port=5
  VDINR_LaneCrossR_flg : Inport  Port=6
  VIFO_InForwardGear_flg : Inport  Port=7
  VIFO_DriverSafetyStatusOk_flg : Inport  Port=8
  VIFO_LatVehicleStatusOk_flg : Inport  Port=9
  VIFO_DriverTurningSignalSwL_flg : Inport  Port=10
  VIFO_DriverTurningSignalSwR_flg : Inport  Port=11
  VPER_CameraStatus_enum : Inport  Port=12
  VDHP_DisableADASFun_flg : Inport  Port=13
  VDHP_DisableLFC_flg : Inport  Port=14
  VFCW_FCWStateHMI_enum : Inport  Port=15
  VAEB_AEBStateHMI_enum : Inport  Port=16
  VLFC_LFCActing_flg : Inport  Port=17
  VLFC_LFCState_enum : Inport  Port=18
  Constant : Constant  OutDataTypeStr=boolean
  LCA_CheckNormal_Conditions : Subsystem
  LCA_Enabled_Conditions : Subsystem
  LCA_LeftAction_Conditions : Subsystem
  LCA_LeftOperationalRecover_Conditions : Subsystem
  LCA_NoADASFailre_Conditions : Subsystem
  LCA_OffRecover_Conditions : Subsystem
  LCA_Operational_Conditions : Subsystem
  LCA_RightAction_Conditions : Subsystem
  LCA_RightOperationalRecover_Conditions : Subsystem
  LCA_StandbyRecover_Conditions : Subsystem
  LCA_TempFailureRecover_Conditions : Subsystem
  LCA_Temporary_Conditions : Subsystem
  VJUD_LCACheckNormal_flg : Outport
  VJUD_LCAEnabledReq_flg : Outport  Port=2
  VJUD_LCAOperationalReq_flg : Outport  Port=3
  VJUD_LCALeftActionReq_flg : Outport  Port=4
  VJUD_LCARightActionReq_flg : Outport  Port=5
  VJUD_LCATempFailureReq_flg : Outport  Port=6
  VJUD_LCANoADASFailure_flg : Outport  Port=7
  VJUD_LCAOffRecover_flg : Outport  Port=8
  VJUD_LCAStandbyRecover_flg : Outport  Port=9
  VJUD_LCALeftOperationalRecover_flg : Outport  Port=10
  VJUD_LCARightOperationalRecover_flg : Outport  Port=11
  VJUD_LCATempFailureRecover_flg : Outport  Port=12
  wires:
  LCA_CheckNormal_Conditions/1(VJUD_LCACheckNormal_flg) -> VJUD_LCACheckNormal_flg/1
  VDINR_KeySwitchStatusValid_flg/1 -> LCA_CheckNormal_Conditions/2(VDINR_KeySwitchStatusValid_flg)
  LCA_Operational_Conditions/1(VJUD_LCAOperationalReq_flg) -> VJUD_LCAOperationalReq_flg/1
  VDINR_KeySwitchStatus_enum/1 -> LCA_CheckNormal_Conditions/1(VDINR_KeySwitchStatus_enum)
  LCA_LeftAction_Conditions/1(VJUD_LCALeftActionReq_flg) -> VJUD_LCALeftActionReq_flg/1
  VIFO_DriverSafetyStatusOk_flg/1 -> LCA_CheckNormal_Conditions/4(VIFO_DriverSafetyStatusOk_flg)
  Constant/1 -> LCA_Enabled_Conditions/1(VDINR_LCAEnableH_flg), [VDINR_LCAEnableH_flg], [VDINR_LCAEnableHValid_flg], LCA_Enabled_Conditions/2(VDINR_LCAEnableHValid_flg)
  LCA_Enabled_Conditions/1(VJUD_LCAEnabledReq_flg) -> VJUD_LCAEnabledReq_flg/1
  VDHP_DisableADASFun_flg/1 -> [VDHP_DisableADASFun_flg], LCA_CheckNormal_Conditions/3(VDHP_DisableADASFun_flg)
  [VDHP_DisableADASFun_flg] -> LCA_Enabled_Conditions/5(VDHP_DisableADASFun_flg)
  VDINR_VehSpd_kph/1 -> [VDINR_VehSpd_kph], LCA_Enabled_Conditions/3(VDINR_VehSpd_kph)
  LCA_Temporary_Conditions/1(VJUD_LCATempFailureReq_flg) -> VJUD_LCATempFailureReq_flg/1
  LCA_NoADASFailre_Conditions/1(VJUD_LCANoADASFailure_flg) -> VJUD_LCANoADASFailure_flg/1
  [VDHP_DisableLFC_flg] -> LCA_NoADASFailre_Conditions/1(VDHP_DisableLFC_flg)
  LCA_OffRecover_Conditions/1(VJUD_LCAOffRecover_flg) -> VJUD_LCAOffRecover_flg/1
  VLFC_LFCActing_flg/1 -> [VLFC_LFCActing_flg], LCA_Operational_Conditions/4(VLFC_LFCActing_flg)
  [VDINR_VehSpd_kph] -> LCA_OffRecover_Conditions/3(VDINR_VehSpd_kph)
  [VDHP_DisableADASFun_flg] -> LCA_OffRecover_Conditions/4(VDHP_DisableADASFun_flg)
  [VDINR_LCAEnableH_flg] -> LCA_OffRecover_Conditions/1(VDINR_LKAEnableH_flg)
  [VDINR_LCAEnableHValid_flg] -> LCA_OffRecover_Conditions/2(VDINR_LKAEnableHValid_flg)
  LCA_StandbyRecover_Conditions/1(VJUD_LCAStandbyRecover_flg) -> VJUD_LCAStandbyRecover_flg/1
  LCA_LeftOperationalRecover_Conditions/1(VJUD_LCALeftOperationalRecover_flg) -> VJUD_LCALeftOperationalRecover_flg/1
  LCA_TempFailureRecover_Conditions/1(VJUD_LCATempFailureRecover_flg) -> VJUD_LCATempFailureRecover_flg/1
  [VDHP_DisableADASFun_flg] -> LCA_TempFailureRecover_Conditions/1(VDHP_DisableADASFun_flg)
  VDHP_DisableLFC_flg/1 -> [VDHP_DisableLFC_flg], LCA_Temporary_Conditions/1(VDHP_DisableLFC_flg)
  VIFO_LatVehicleStatusOk_flg/1 -> LCA_CheckNormal_Conditions/5(VIFO_LatVehicleStatusOk_flg)
  VPER_CameraStatus_enum/1 -> LCA_CheckNormal_Conditions/6(VPER_CameraStatus_enum)
  VIFO_InForwardGear_flg/1 -> [VIFO_InForwardGear_flg], LCA_Enabled_Conditions/4(VIFO_InForwardGear_flg)
  [VIFO_InForwardGear_flg] -> LCA_OffRecover_Conditions/5(VIFO_InForwardGear_flg)
  VFCW_FCWStateHMI_enum/1 -> [VFCW_FCWStateHMI_enum], LCA_Operational_Conditions/1(VFCW_FCWStateHMI_enum)
  VAEB_AEBStateHMI_enum/1 -> [VAEB_AEBStateHMI_enum], LCA_Operational_Conditions/2(VAEB_AEBStateHMI_enum)
  LCA_RightOperationalRecover_Conditions/1(VJUD_LCARightOperationalRecover_flg) -> VJUD_LCARightOperationalRecover_flg/1
  [VFCW_FCWStateHMI_enum] -> LCA_StandbyRecover_Conditions/1(VFCW_FCWStateHMI_enum)
  [VAEB_AEBStateHMI_enum] -> LCA_StandbyRecover_Conditions/2(VAEB_AEBStateHMI_enum)
  VLFC_LFCState_enum/1 -> LCA_Operational_Conditions/3(VLFC_LFCState_enum)
  LCA_RightAction_Conditions/1(VJUD_LCARightActionReq_flg) -> VJUD_LCARightActionReq_flg/1
  [VLFC_LFCActing_flg] -> LCA_StandbyRecover_Conditions/3(VLFC_LFCActing_flg)
  [VIFO_DriverTurningSignalSwL_flg] -> LCA_LeftOperationalRecover_Conditions/1(VIFO_DriverTurningSignalSwL_flg)
  [VIFO_DriverTurningSignalSwR_flg] -> LCA_RightOperationalRecover_Conditions/1(VIFO_DriverTurningSignalSwR_flg)
  VDINR_EPSLFCStatus_enum/1 -> [VDINR_EPSLFCStatus_enum], LCA_Temporary_Conditions/2(VDINR_EPSLFCStatus_enum)
  [VDINR_EPSLFCStatus_enum] -> LCA_TempFailureRecover_Conditions/2(VDINR_EPSLFCStatus_enum)
  VDINR_LaneCrossL_flg/1 -> LCA_LeftOperationalRecover_Conditions/2(VDINR_LaneCrossL_flg)
  VDINR_LaneCrossR_flg/1 -> LCA_RightOperationalRecover_Conditions/2(VDINR_LaneCrossR_flg)
  VIFO_DriverTurningSignalSwL_flg/1 -> [VIFO_DriverTurningSignalSwL_flg], LCA_LeftAction_Conditions/1(VIFO_DriverTurningSignalSwL_flg)
  VIFO_DriverTurningSignalSwR_flg/1 -> LCA_RightAction_Conditions/1(VIFO_DriverTurningSignalSwR_flg), [VIFO_DriverTurningSignalSwR_flg]

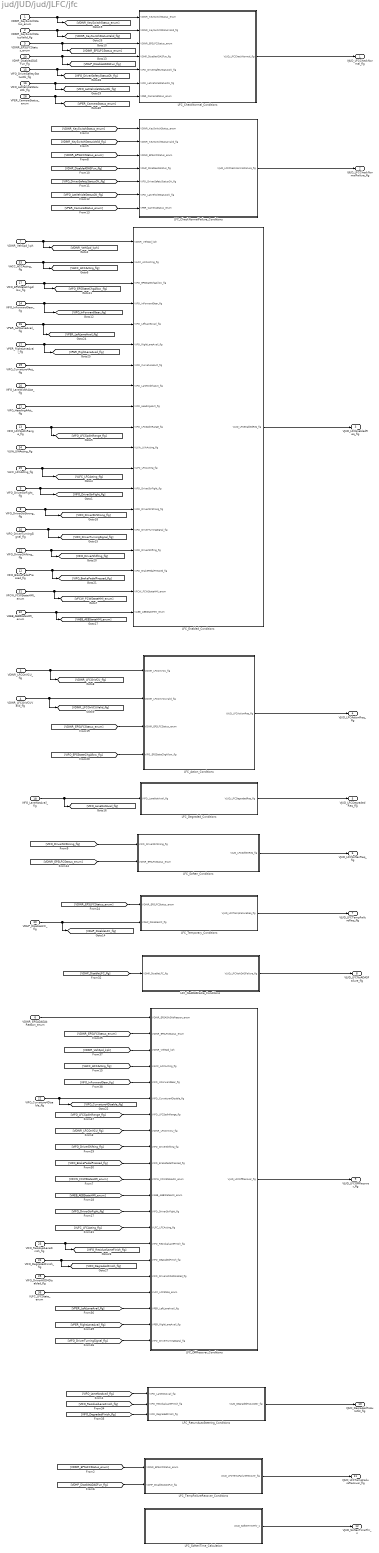
== system jud/JUD/jud/JLFC/jfc ==
  VDINR_KeySwitchStatus_enum : Inport
  VDINR_KeySwitchStatusValid_flg : Inport  Port=2
  VDINR_LFCOnVCU_flg : Inport  Port=3
  VDINR_LFCOnVCUValid_flg : Inport  Port=4
  VDINR_EPSLFCStatus_enum : Inport  Port=5
  VDINR_EPSADASAbReason_enum : Inport  Port=6
  VDINR_VehSpd_kph : Inport  Port=7
  VIFO_DriverStrStrong_flg : Inport  Port=8
  VIFO_DriverStrFight_flg : Inport  Port=9
  VIFO_DriverTurningSignal_flg : Inport  Port=10
  VIFO_DriverShifting_flg : Inport  Port=11
  VIFO_BrakePedalPressed_flg : Inport  Port=12
  "VIFO_LFCSpdInRange_flg " : Inport  Port=13
  VIFO_InForwardGear_fig : Inport  Port=14
  VIFO_DriverSafetyStatusOk_flg : Inport  Port=15
  VIFO_LatVehicleStatusOk_flg : Inport  Port=16
  VIFO_EPSStateChgAllow_flg : Inport  Port=17
  VIFO_LaneNotAvail_fig : Inport  Port=18
  VIFO_Curvature4Act_flg : Inport  Port=19
  VIFO_LaneWidth4Act_flg : Inport  Port=20
  VIFO_Heading4Act_flg : Inport  Port=21
  VIFO_Curvature4Disable_flg : Inport  Port=22
  VIFO_ResidualLaneFinish_flg : Inport  Port=23
  VIFO_DegradedFinish_flg : Inport  Port=24
  VIFO_DriverHOD4Disabled_flg : Inport  Port=25
  VPER_LeftLaneAvail_flg : Inport  Port=26
  VPER_RightLaneAvail_flg : Inport  Port=27
  VPER_CameraStatus_enum : Inport  Port=28
  VDHP_DisableADASFun_flg : Inport  Port=29
  VDHP_DisableLFC_flg : Inport  Port=30
  VFCW_FCWStateHMI_enum : Inport  Port=31
  VAEB_AEBStateHMI_enum : Inport  Port=32
  VACC_ACCActing_flg : Inport  Port=33
  VLKA_LKAActing_flg : Inport  Port=34
  VLFC_LFCActing_flg : Inport  Port=35
  VLFC_LFCState_enum : Inport  Port=36
  LFC_Action_Conditions : Subsystem
  LFC_CheckNormalFailure_Conditions : Subsystem
  LFC_CheckNormal_Conditions : Subsystem
  LFC_Degraded_Conditions : Subsystem
  LFC_Enabled_Conditions : Subsystem
  LFC_NoADASFailre_Conditions : Subsystem
  LFC_OffRecover_Conditions : Subsystem
  LFC_ReturnAutoSteering_Conditions : Subsystem
  LFC_SoftenTime_Calculation : Subsystem
  LFC_Soften_Conditions : Subsystem
  LFC_TempFailureRecover_Conditions : Subsystem
  LFC_Temporary_Conditions : Subsystem
  VJUD_LFCCheckNormal_flg : Outport
  VJUD_LFCCheckNormalFailure_flg : Outport  Port=2
  VJUD_LFCEnabledReq_flg : Outport  Port=3
  VJUD_LFCActionReq_flg : Outport  Port=4
  VJUD_LFCDegradedReq_flg : Outport  Port=5
  VJUD_LFCSoftenReq_flg : Outport  Port=6
  VJUD_LFCTempFailureReq_flg : Outport  Port=7
  VJUD_LFCNoADASFailure_flg : Outport  Port=8
  VJUD_LFCOffRecover_flg : Outport  Port=9
  VJUD_DegradedToAutoStr_flg : Outport  Port=10
  VJUD_LFCTempFailureRecover_flg : Outport  Port=11
  VJUD_SoftenTimeThr_s : Outport  Port=12
  wires:
  LFC_CheckNormal_Conditions/1(VJUD_LFCCheckNormal_flg) -> VJUD_LFCCheckNormal_flg/1
  VDINR_KeySwitchStatusValid_flg/1 -> [VDINR_KeySwitchStatusValid_flg], LFC_CheckNormal_Conditions/2(VDINR_KeySwitchStatusValid_flg)
  LFC_Action_Conditions/1(VJUD_LFCActionReq_flg) -> VJUD_LFCActionReq_flg/1
  VDINR_KeySwitchStatus_enum/1 -> [VDINR_KeySwitchStatus_enum], LFC_CheckNormal_Conditions/1(VDINR_KeySwitchStatus_enum)
  LFC_SoftenTime_Calculation/1(VJUD_SoftenTimeThr_s) -> VJUD_SoftenTimeThr_s/1
  VIFO_DriverSafetyStatusOk_flg/1 -> [VIFO_DriverSafetyStatusOk_flg], LFC_CheckNormal_Conditions/5(VIFO_DriverSafetyStatusOk_flg)
  VACC_ACCActing_flg/1 -> [VACC_ACCActing_flg], LFC_Enabled_Conditions/2(VACC_ACCActing_flg)
  LFC_Enabled_Conditions/1(VJUD_LFCEnabledReq_flg) -> VJUD_LFCEnabledReq_flg/1
  VDINR_LFCOnVCU_flg/1 -> LFC_Action_Conditions/1(VDINR_LFCOnVCU_flg), [VDINR_LFCOnVCU_flg]
  VDINR_LFCOnVCUValid_flg/1 -> [VDINR_LFCOnVCUValid_flg], LFC_Action_Conditions/2(VDINR_LFCOnVCUValid_flg)
  LFC_Degraded_Conditions/1(VJUD_LFCDegradedReq_flg) -> VJUD_LFCDegradedReq_flg/1
  LFC_Temporary_Conditions/1(VJUD_LFCTempFailureReq_flg) -> VJUD_LFCTempFailureReq_flg/1
  LFC_NoADASFailre_Conditions/1(VJUD_LFCNoADASFailure_flg) -> VJUD_LFCNoADASFailure_flg/1
  [VACC_ACCActing_flg] -> LFC_OffRecover_Conditions/4(VACC_ACCActing_flg)
  LFC_OffRecover_Conditions/1(VJUD_LFCOffRecover_flg) -> VJUD_LFCOffRecover_flg/1
  [VIFO_EPSStateChgAllow_flg] -> LFC_Action_Conditions/4(VIFO_EPSStateChgAllow_flg)
  [VDINR_EPSLFCStatus_enum] -> LFC_Temporary_Conditions/1(VDINR_EPSLFCStatus_enum)
  VDHP_DisableADASFun_flg/1 -> [VDHP_DisableADASFun_flg], LFC_CheckNormal_Conditions/4(VDHP_DisableADASFun_flg)
  VIFO_EPSStateChgAllow_flg/1 -> [VIFO_EPSStateChgAllow_flg], LFC_Enabled_Conditions/3(VIFO_EPSStateChgAllow_flg)
  VDINR_EPSLFCStatus_enum/1 -> LFC_CheckNormal_Conditions/3(VDINR_EPSLFCStatus_enum), [VDINR_EPSLFCStatus_enum]
  VDHP_DisableLFC_flg/1 -> [VDHP_DisableLFC_flg], LFC_Temporary_Conditions/2(VDHP_DisableLFC_flg)
  [VDHP_DisableLFC_flg] -> LFC_NoADASFailre_Conditions/1(VDHP_DisableLFC_flg)
  VDINR_EPSADASAbReason_enum/1 -> LFC_OffRecover_Conditions/1(VDINR_EPSADASAbReason_enum)
  [VDINR_EPSLFCStatus_enum] -> LFC_OffRecover_Conditions/2(VDINR_EPSLFCStatus_enum)
  [VDINR_EPSLFCStatus_enum] -> LFC_TempFailureRecover_Conditions/1(VDINR_EPSLFCStatus_enum)
  [VDHP_DisableADASFun_flg] -> LFC_TempFailureRecover_Conditions/2(VDHP_DisableADASFun_flg)
  LFC_TempFailureRecover_Conditions/1(VJUD_LFCTempFailureRecover_flg) -> VJUD_LFCTempFailureRecover_flg/1
  VDINR_VehSpd_kph/1 -> [VDINR_VehSpd_kph], LFC_Enabled_Conditions/1(VDINR_VehSpd_kph)
  VIFO_InForwardGear_fig/1 -> [VIFO_InForwardGear_fig], LFC_Enabled_Conditions/4("VIFO_InForwardGear_flg ")
  [VIFO_InForwardGear_fig] -> LFC_OffRecover_Conditions/5(VIFO_InForwardGear_flg)
  [VDINR_VehSpd_kph] -> LFC_OffRecover_Conditions/3(VDINR_VehSpd_kph)
  VIFO_LatVehicleStatusOk_flg/1 -> [VIFO_LatVehicleStatusOk_flg], LFC_CheckNormal_Conditions/6(VIFO_LatVehicleStatusOk_flg)
  "VIFO_LFCSpdInRange_flg "/1 -> [VIFO_LFCSpdInRange_flg], LFC_Enabled_Conditions/10(VIFO_LFCSpdInRange_flg)
  VPER_CameraStatus_enum/1 -> [VPER_CameraStatus_enum], LFC_CheckNormal_Conditions/7(VPER_CameraStatus_enum)
  VLFC_LFCActing_flg/1 -> LFC_Enabled_Conditions/12(VLFC_LFCActing_flg), [VLFC_LFCActing_flg]
  VIFO_LaneNotAvail_fig/1 -> [VIFO_LaneNotAvail_flg], LFC_Degraded_Conditions/1(VIFO_LaneNotAvail_flg)
  LFC_ReturnAutoSteering_Conditions/1(VJUD_DegradedToAutoStr_flg) -> VJUD_DegradedToAutoStr_flg/1
  [VIFO_LaneNotAvail_flg] -> LFC_ReturnAutoSteering_Conditions/1(VIFO_LaneNotAvail_flg)
  LFC_Soften_Conditions/1(VJUD_LFCSoftenReq_flg) -> VJUD_LFCSoftenReq_flg/1
  VIFO_DriverStrFight_flg/1 -> [VIFO_DriverStrFight_flg], LFC_Enabled_Conditions/13(VIFO_DriverStrFight_flg)
  VIFO_DriverStrStrong_flg/1 -> [VIFO_DriverStrStrong_flg], LFC_Enabled_Conditions/14(VIFO_DriverStrStrong_flg)
  [VIFO_DriverStrStrong_flg] -> LFC_Soften_Conditions/1(VIFO_DriverStrStrong_flg)
  [VDINR_EPSLFCStatus_enum] -> LFC_Action_Conditions/3(VDINR_EPSLFCStatus_enum)
  VPER_LeftLaneAvail_flg/1 -> [VPER_LeftLaneAvail_flg], LFC_Enabled_Conditions/5(VIFO_LeftLaneAvail_flg)
  VPER_RightLaneAvail_flg/1 -> [VPER_RightLaneAvail_flg], LFC_Enabled_Conditions/6(VIFO_RightLaneAvail_flg)
  VIFO_Curvature4Act_flg/1 -> LFC_Enabled_Conditions/7(VIFO_Curvature4Act_flg)
  VIFO_LaneWidth4Act_flg/1 -> LFC_Enabled_Conditions/8(VIFO_LaneWidth4Act_flg)
  VIFO_Heading4Act_flg/1 -> LFC_Enabled_Conditions/9(VIFO_Heading4Act_flg)
  VLKA_LKAActing_flg/1 -> LFC_Enabled_Conditions/11(VLKA_LKAActing_flg)
  VIFO_DriverTurningSignal_flg/1 -> [VIFO_DriverTurningSignal_flg], LFC_Enabled_Conditions/15(VIFO_DriverTurningSignal_flg)
  VIFO_DriverShifting_flg/1 -> LFC_Enabled_Conditions/16(VIFO_DriverShifting_flg), [VIFO_DriverShifting_flg]
  VIFO_BrakePedalPressed_flg/1 -> LFC_Enabled_Conditions/17(VIFO_BrakePedalPressed_flg), [VIFO_BrakePedalPressed_flg]
  VFCW_FCWStateHMI_enum/1 -> [VFCW_FCWStateHMI_enum], LFC_Enabled_Conditions/18(VFCW_FCWStateHMI_enum)
  VAEB_AEBStateHMI_enum/1 -> [VAEB_AEBStateHMI_enum], LFC_Enabled_Conditions/19(VAEB_AEBStateHMI_enum)
  VIFO_Curvature4Disable_flg/1 -> [VIFO_Curvature4Disable_flg], LFC_OffRecover_Conditions/6(VIFO_Curvature4Disable_flg)
  [VIFO_LFCSpdInRange_flg] -> LFC_OffRecover_Conditions/7(VIFO_LFCSpdInRange_flg)
  [VDINR_LFCOnVCU_flg] -> LFC_OffRecover_Conditions/8(VDINR_LFCOnVCU_flg)
  [VIFO_DriverShifting_flg] -> LFC_OffRecover_Conditions/9(VIFO_DriverShifting_flg)
  [VIFO_BrakePedalPressed_flg] -> LFC_OffRecover_Conditions/10(VIFO_BrakePedalPressed_flg)
  [VIFO_DriverStrFight_flg] -> LFC_OffRecover_Conditions/13(VIFO_DriverStrFight_flg)
  [VAEB_AEBStateHMI_enum] -> LFC_OffRecover_Conditions/12(VAEB_AEBStateHMI_enum)
  [VFCW_FCWStateHMI_enum] -> LFC_OffRecover_Conditions/11(VFCW_FCWStateHMI_enum)
  [VLFC_LFCActing_flg] -> LFC_OffRecover_Conditions/14(VLFC_LFCActing_flg)
  VIFO_DegradedFinish_flg/1 -> [VIFO_DegradedFinish_flg], LFC_OffRecover_Conditions/16(VIFO_DegradedFinish_flg)
  VIFO_ResidualLaneFinish_flg/1 -> [VIFO_ResidualLaneFinish_flg], LFC_OffRecover_Conditions/15(VIFO_ResidualLaneFinish_flg)
  [VIFO_ResidualLaneFinish_flg] -> LFC_ReturnAutoSteering_Conditions/2(VIFO_ResidualLaneFinish_flg)
  [VIFO_DegradedFinish_flg] -> LFC_ReturnAutoSteering_Conditions/3(VIFO_DegradedFinish_flg)
  VIFO_DriverHOD4Disabled_flg/1 -> LFC_OffRecover_Conditions/17(VIFO_DriverHOD4Disabled_flg)
  VLFC_LFCState_enum/1 -> LFC_OffRecover_Conditions/18(VLFC_LFCState_enum)
  [VPER_LeftLaneAvail_flg] -> LFC_OffRecover_Conditions/19(VPER_LeftLaneAvail_flg)
  [VPER_RightLaneAvail_flg] -> LFC_OffRecover_Conditions/20(VPER_RightLaneAvail_flg)
  [VDINR_KeySwitchStatus_enum] -> LFC_CheckNormalFailure_Conditions/1(VDINR_KeySwitchStatus_enum)
  [VDINR_KeySwitchStatusValid_flg] -> LFC_CheckNormalFailure_Conditions/2(VDINR_KeySwitchStatusValid_flg)
  [VDINR_EPSLFCStatus_enum] -> LFC_CheckNormalFailure_Conditions/3(VDINR_EPSLFCStatus_enum)
  [VDHP_DisableADASFun_flg] -> LFC_CheckNormalFailure_Conditions/4(VDHP_DisableADASFun_flg)
  [VIFO_DriverSafetyStatusOk_flg] -> LFC_CheckNormalFailure_Conditions/5(VIFO_DriverSafetyStatusOk_flg)
  [VIFO_LatVehicleStatusOk_flg] -> LFC_CheckNormalFailure_Conditions/6(VIFO_LatVehicleStatusOk_flg)
  [VPER_CameraStatus_enum] -> LFC_CheckNormalFailure_Conditions/7(VPER_CameraStatus_enum)
  LFC_CheckNormalFailure_Conditions/1(VJUD_LFCCheckNormalFailure_flg) -> VJUD_LFCCheckNormalFailure_flg/1
  [VDINR_EPSLFCStatus_enum] -> LFC_Soften_Conditions/2(VDINR_EPSLFCStatus_enum)
  [VIFO_DriverTurningSignal_flg] -> LFC_OffRecover_Conditions/21(VIFO_DriverTurningSignal_flg)
